simulink model "suspension_rig_cosimulation"  (R2021b)
settings: Solver=ode45  StartTime=0.0  StopTime=10  FixedStep=0.01  RelTol=1e-3  EnableMultiTasking=on
libraries: simulink x5, instrumentlib x2, simulink_extras x1
settings Model: PacingRate=11  Creator=tasora  LastModifiedBy=Trevor
settings SolverCC: AlgebraicLoopSolver=TrustRegion
settings DataIOCC: LimitDataPoints=on  SaveFormat=Array  SignalLoggingSaveFormat=ModelDataLogs  ReturnWorkspaceOutputs=off
settings OptimizationCC: ExpressionDepthLimit=2147483647  LifeSpan=inf
settings DebuggingCC: UnderspecifiedInitializationDetection=Classic  MergeDetectMultiDrivingBlocksExec=none  SolverPrmCheckMsg=warning  FcnCallInpInsideContextMsg=warning  StateNameClashWarn=warning  SFUnexpectedBacktrackingDiag=warning  SFNoUnconditionalDefaultTransitionDiag=warning  SFExecutionAtInitializationDiag=none  SFMachineParentedDataDiag=warning  ArithmeticOperatorsInVariantConditions=warning
settings HardwareCC: ProdBitPerPointer=32  ProdBitPerSizeT=32  ProdBitPerPtrDiffT=32  ProdLargestAtomicFloat=None  ProdIntDivRoundTo=Undefined  ProdEndianess=Unspecified  ProdWordSize=32  ProdHWDeviceType=32-bit Generic
settings ModelReferenceCC: PropagateSignalLabelsOutOfModel=off
settings SFSimCC: SimUseLocalCustomCode=off  CustomCodeUndefinedFunction=UseInterfaceOnly
settings RTWCC: RTWUseLocalCustomCode=off
settings CodeAppCC: StateflowObjectComments=on
settings GRTTargetCC: TargetLangStandard=C89/C90 (ANSI)  CombineOutputUpdateFcns=off  GRTInterface=on
settings ConfigComp: CovMetricSettings=dw  CovSaveCumulativeToWorkspaceVar=on  CovSaveSingleToWorkspaceVar=on  CovExternalEMLEnable=off

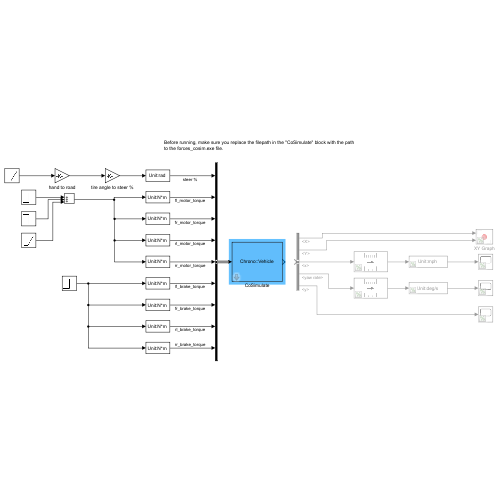
[thumbnail: Simulink's stored preview of the top-level diagram]
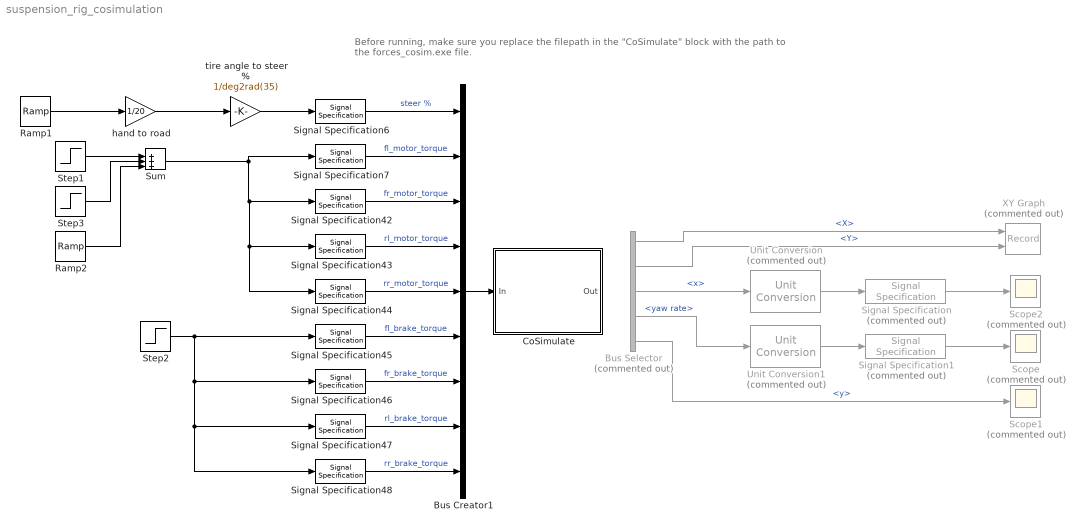
== system suspension_rig_cosimulation ==
  note: Before running, make sure you replace the filepath in the "CoSimulate" block with the path to the forces_cosim.exe file.
  Bus Creator1 : BusCreator  Inputs=9
  Bus Selector : BusSelector  Commented=on  OutputSignals=global frame.position.X,global frame.position.Y,chassis frame.velocity.x,chassis frame.rotational velocity.yaw rate,chassis frame.acceleration.y
  CoSimulate : Subsystem  Description=|  mask{com_step=1e-2, tcp_data_size=16, host_name=localhost, tcp_port=50009, tcp_timeout=5, exec_path=C:\Users\Trevor\Project Chrono\chrono_simulink_cosim\build\Release\cosim_suspensionrig.exe}
      | This block can be used to exchange data with Chrono::Engine.                                                                                      
      | A Chrono::Engine program with a running ChCosimulation inferface must be started, it will work as a server; then the Simulink program must be run.
      | Note! check that the dimensions of the exchanged vectors do match!
      mask prompts: com_step "Communication step size"; tcp_data_size "N. of scalars received from C::E (as block output)"; host_name "TCP host name (ex. 'localhost', or 'www.myhost.com')"; tcp_port "TCP port (ex. 50007)"; tcp_timeout "TCP timeout (seconds)"; exec_path "Executable Path:"
      mask init:
      | block_receive = [gcb, '/TCP Receive'];
      | set_param(block_receive, 'SampleTime', num2str(com_step));
      | set_param(block_receive, 'Host', host_name);
      | set_param(block_receive, 'Port', num2str(tcp_port));
      | set_param(block_receive, 'DataSize', num2str(tcp_data_size+1));
      | set_param(block_receive, 'Timeout', num2str(tcp_timeout));
      | block_send = [gcb, '/TCP Send'];
      | set_param(block_send, 'Host', host_name);
      | set_param(block_send, 'Port', num2str(tcp_port));
      | 
      | % Set the executable extension depending on the OS.
      | if ismac
      |     error("This model cannot run on Mac devices");
      | elseif isunix
      |     extension = "";
      | elseif ispc
      |     extension = ".exe";
      | else
      |     error("Platform not supported")
      | end
      | 
      | % Run Chrono::Vehicle executable.
      | if ~isstring(exec_path)
      |     exec_path = string(exec_path);
      | end
      | if ~isfile(exec_path)
      |     error("The file: '%s', cannot be found.",exec_path);
      | end
      | system(['"', char(exec_path),'" ',num2str(tcp_port),' &']);
      | 
      | % Wait for the executable to establish the TCP server.
      | pause(1.0);
      mask DialogControl Control2 Prompt: Enter below the filepath to the Chrono::Vehicle executable you want to run. In Windows, you can do this:
      mask DialogControl Control4 Prompt: 1. Locate the ".exe" file in File Explorer.
      mask DialogControl Control5 Prompt: 2. Right-click on the executable (ends with ".exe") and select "Copy as Path".
      mask DialogControl Control3 Prompt: 3. Paste the path below.
      mask DialogControl file_path Prompt: Choose cosim executable
      mask DialogControl file_path Callback:
      | [file,path] = uigetfile("*.exe");
      | file_path = string([path,file]);
      | set_param(gcb,'exec_path',file_path);
      mask Display: disp('Chrono::Vehicle')
  Ramp1 : simulink/Sources/Ramp  slope=-deg2rad(13)  start=10  InitialOutput=0
  Ramp2 : simulink/Sources/Ramp  slope=10  start=9.5  InitialOutput=0
  Scope : Scope  Commented=on
  Scope1 : Scope  Commented=on
  Scope2 : Scope  Commented=on
  Signal Specification : SignalSpecification  Commented=on  Unit=mph
  Signal Specification1 : SignalSpecification  Commented=on  Unit=deg/s
  Signal Specification{7,42..48} (8 alike) : SignalSpecification  Unit=N*m
  Signal Specification6 : SignalSpecification  Unit=rad
  Step1 : Step  Time=3  After=500  SampleTime=0
  Step2 : Step  Time=40  After=2000  SampleTime=0
  Step3 : Step  Time=9.5  After=-490  SampleTime=0
  Sum : Sum  Inputs=|+++
  Unit Conversion : UnitConversion  Commented=on
  Unit Conversion1 : UnitConversion  Commented=on
  XY Graph : Record  Commented=on  FileSettingsInternal="{\"entries\":[{\"content\":{\"excelSettings\":{\"content\":{},\"type\":\"Streamout.ExcelSettings\"}},\"type\":\"Streamout.FileSettingStorage\",\"uuid\":\"918d6b58-b81c-43a7-aac3-45bd64a5f4ef\"}],\"packageUris\":[\"http://schema.mathworks.com/mf0/streamout_blocks/R2020a\"],\"version\":\"1.0\"}"  Layout=[1 1]  SignalsInternal="{\"entries\":[{\"content\":{\"signals\":[]},\"type\":\"RecordBlkView.InputSignals\",\"uuid\":\"825a583e-bb3f-4325-a404-8858829500c0\"}],\"packageUris\":[\"http://schema.mathworks.com/mf0/streamout_blocks/R2020a\"],\"version\":\"1.0\"}"  VisualizationBindings="{\"xyplotplugin\":{\"info\":[{\"series\":[],\"subplotID\":1}]}}"  CompatibilityTag=XY
  hand to road : Gain  Gain=1/20
  tire angle to steer % : Gain  Gain=1/deg2rad(35)
  wires:
  Bus Creator1/1 -> CoSimulate/1(In)
  Bus Selector/1 -> XY Graph/1  "<X>"
  Bus Selector/2 -> XY Graph/2  "<Y>"
  Bus Selector/4 -> Unit Conversion1/1  "<yaw rate>"
  Bus Selector/5 -> Scope1/1  "<y>"
  Bus Selector/3 -> Unit Conversion/1  "<x>"
  Unit Conversion/1 -> Signal Specification/1
  Signal Specification/1 -> Scope2/1
  Unit Conversion1/1 -> Signal Specification1/1
  Signal Specification1/1 -> Scope/1
  Ramp2/1 -> Sum/3
  Step1/1 -> Sum/1
  Ramp1/1 -> hand to road/1
  hand to road/1 -> tire angle to steer %/1
  Signal Specification44/1 -> Bus Creator1/5  "rr_motor_torque"
  tire angle to steer %/1 -> Signal Specification6/1
  Signal Specification43/1 -> Bus Creator1/4  "rl_motor_torque"
  Signal Specification7/1 -> Bus Creator1/2  "fl_motor_torque"
  Signal Specification42/1 -> Bus Creator1/3  "fr_motor_torque"
  Signal Specification45/1 -> Bus Creator1/6  "fl_brake_torque"
  Signal Specification6/1 -> Bus Creator1/1  "steer %"
  Signal Specification46/1 -> Bus Creator1/7  "fr_brake_torque"
  Step2/1 -> Signal Specification45/1, Signal Specification46/1, Signal Specification48/1, Signal Specification47/1
  Signal Specification48/1 -> Bus Creator1/9  "rr_brake_torque"
  Signal Specification47/1 -> Bus Creator1/8  "rl_brake_torque"
  Step3/1 -> Sum/2
  Sum/1 -> Signal Specification7/1, Signal Specification44/1, Signal Specification43/1, Signal Specification42/1

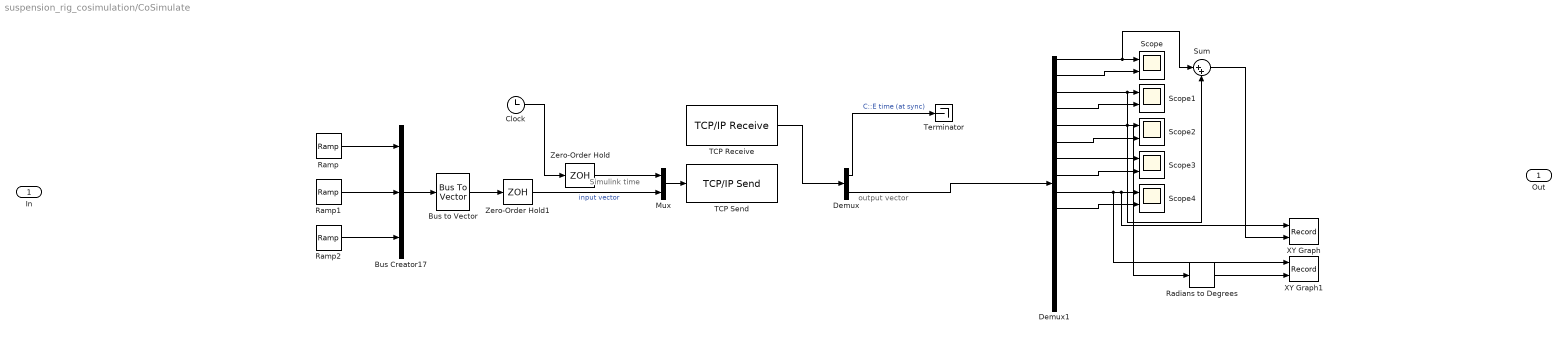
== system suspension_rig_cosimulation/CoSimulate ==
  note: output vector
  note: Simulink time
  In : Inport
  Bus Creator17 : BusCreator  Inputs=3
  Bus to Vector : BusToVector
  Clock : Clock
  Demux : Demux  Outputs=[1 -1]
  Demux1 : Demux  Outputs=16
  Mux : Mux  Inputs=2
  Radians to Degrees : simulink_extras/Transformations/Radians to Degrees
  Ramp : simulink/Sources/Ramp  slope=0  start=0  InitialOutput=0
  Ramp1 : simulink/Sources/Ramp  slope=0.2  start=0  InitialOutput=-1
  Ramp2 : simulink/Sources/Ramp  slope=0.2  start=0  InitialOutput=-1
  Scope{,1..4} (5 alike) : Scope  NumInputPorts=2
  Sum : Sum  Inputs=|++
  TCP Receive : instrumentlib/TCP//IP Receive  Priority=2  Host=localhost  Port=50009  DataSize=17  DataType=double  ASCIIFormatting=%f  Terminator=LF  CustomTerminator=10  ByteOrder=little-endian  EnableBlockingMode=on  Timeout=5  SampleTime=0.01  SimulateUsing=Interpreted execution
  TCP Send : instrumentlib/TCP//IP Send  Priority=3  Host=localhost  Port=50009  ByteOrder=little-endian  EnableBlockingMode=off  Timeout=10  TransferDelay=on  SimulateUsing=Interpreted execution
  Terminator : Terminator
  XY Graph : Record  FileSettingsInternal="{\"entries\":[{\"content\":{\"excelSettings\":{\"content\":{},\"type\":\"Streamout.ExcelSettings\"}},\"type\":\"Streamout.FileSettingStorage\",\"uuid\":\"c42a29d6-a723-4289-96b4-a2cca099133b\"}],\"packageUris\":[\"http://schema.mathworks.com/mf0/streamout_blocks/R2020a\"],\"version\":\"1.0\"}"  Layout=[1 1]  SignalsInternal="{\"entries\":[{\"content\":{\"signals\":[{\"content\":{\"blockPath\":[\"suspension_rig_cosimulation/CoSimulate/XY Graph\"],\"channel\":[],\"dimensions\":[1,1],\"domain\":\"suspension_rig_cosimulation/CoSimulate/XY Graph\",\"lineColor\":\"#a2142f\",\"plots\":[],\"port\":1,\"sid\":[\"\"],\"signalID\":45527,\"signalName\":\"Demux1:9\"},\"type\":\"RecordBlkView.Signal\",\"uuid\":\"382ebe2f-5953-4c3d-b8b2-6b4942b9b3dc\"},{\"content\":{\"blockPath\":[\"suspension_rig_cosimulation/CoSimulate/XY Graph\"],\"channel\":[],\"dimensions\":[1,1],\"domain\":\"suspension_rig_cosimulation/CoSimulate/XY Graph\",\"lineColor\":\"#139fff\",\"plots\":[],\"port\":2,\"sid\":[\"\"],\"signalID\":45531,\"signalName\":\"Sum\"},\"type\":\"RecordBlkView.Signal\",\"uuid\":\"1248ef68-174a-4df7-9daa-54e234e1ff71\"}]},\"type\":\"RecordBlkView.InputSignals\",\"uuid\":\"0179d33f-e8d5-4601-95fc-4a47f65f2947\"}],\"packageUris\":[\"http://schema.mathworks.com/mf0/streamout_blocks/R2020a\"],\"version\":\"1.0\"}"  VisualizationBindings="{\"xyplotplugin\":{\"info\":[{\"series\":[{\"bindingParametersList\":[{\"parameter\":\"X-Axis\",\"signalID\":45527,\"signalName\":\"Demux1:9\"},{\"parameter\":\"Y-Axis\",\"signalID\":45531,\"signalName\":\"Sum\"}],\"seriesID\":4984}],\"subplotID\":1}]}}"  CompatibilityTag=XY
  XY Graph1 : Record  FileSettingsInternal="{\"entries\":[{\"content\":{\"excelSettings\":{\"content\":{},\"type\":\"Streamout.ExcelSettings\"}},\"type\":\"Streamout.FileSettingStorage\",\"uuid\":\"61cc620a-e358-4595-980b-47bd051c2f1a\"}],\"packageUris\":[\"http://schema.mathworks.com/mf0/streamout_blocks/R2020a\"],\"version\":\"1.0\"}"  Layout=[1 1]  SignalsInternal="{\"entries\":[{\"content\":{\"signals\":[{\"content\":{\"blockPath\":[\"suspension_rig_cosimulation/CoSimulate/XY Graph1\"],\"channel\":[],\"dimensions\":[1,1],\"domain\":\"suspension_rig_cosimulation/CoSimulate/XY Graph1\",\"lineColor\":\"#a2142f\",\"plots\":[],\"port\":1,\"sid\":[\"\"],\"signalID\":45535,\"signalName\":\"Demux1:9\"},\"type\":\"RecordBlkView.Signal\",\"uuid\":\"fd3578e4-31df-4f63-a0b1-c924a1c19dd5\"},{\"content\":{\"blockPath\":[\"suspension_rig_cosimulation/CoSimulate/XY Graph1\"],\"channel\":[],\"dimensions\":[1,1],\"domain\":\"suspension_rig_cosimulation/CoSimulate/XY Graph1\",\"lineColor\":\"#139fff\",\"plots\":[],\"port\":2,\"sid\":[\"\"],\"signalID\":45539,\"signalName\":\"Radians\\nto Degrees\"},\"type\":\"RecordBlkView.Signal\",\"uuid\":\"7a3ece93-7a64-46ff-9a4a-2255d9852275\"}]},\"type\":\"RecordBlkView.InputSignals\",\"uuid\":\"4b1f62b5-0216-408a-8ebb-b9535f346377\"}],\"packageUris\":[\"http://schema.mathworks.com/mf0/streamout_blocks/R2020a\"],\"version\":\"1.0\"}"  VisualizationBindings="{\"xyplotplugin\":{\"info\":[{\"series\":[{\"bindingParametersList\":[{\"parameter\":\"X-Axis\",\"signalID\":45535,\"signalName\":\"Demux1:9\"},{\"parameter\":\"Y-Axis\",\"signalID\":45539,\"signalName\":\"Radians\\nto Degrees\"}],\"seriesID\":47074}],\"subplotID\":1}]}}"  CompatibilityTag=XY
  Zero-Order Hold : ZeroOrderHold  SampleTime=com_step
  Zero-Order Hold1 : ZeroOrderHold  SampleTime=com_step
  Out : Outport
  wires:
  Zero-Order Hold/1 -> Mux/1
  Zero-Order Hold1/1 -> Mux/2  "input vector"
  Mux/1 -> TCP Send/1
  Clock/1 -> Zero-Order Hold/1
  TCP Receive/1 -> Demux/1
  Demux/1 -> Terminator/1  "C::E time (at sync)"
  Bus to Vector/1 -> Zero-Order Hold1/1
  Bus Creator17/1 -> Bus to Vector/1
  Demux/2 -> Demux1/1
  Demux1/1 -> Sum/1, Scope/1
  Ramp/1 -> Bus Creator17/1
  Ramp1/1 -> Bus Creator17/2
  Ramp2/1 -> Bus Creator17/3
  Demux1/2 -> Scope/2
  Demux1/3 -> Sum/2, Scope1/1
  Demux1/4 -> Scope1/2
  Demux1/5 -> Radians to Degrees/1, Scope2/1
  Demux1/6 -> Scope2/2
  Demux1/7 -> Scope3/1
  Demux1/8 -> Scope3/2
  Demux1/9 -> XY Graph1/1, XY Graph/1, Scope4/1
  Demux1/10 -> Scope4/2
  Sum/1 -> XY Graph/2
  Radians to Degrees/1 -> XY Graph1/2
